simulink model "lqr_hovering"  (R2017a)
settings: Solver=ode5  StartTime=0.0  StopTime=50  FixedStep=Ts  RelTol=1e-3  EnableMultiTasking=on
undefined symbols (not defined in the file or in its folder): B_ENU_inv, gra, Ki_lqr, KT, Kx_lqr, mass
settings Model: Creator=dtnguyen  LastModifiedBy=ducnguyen
settings DataIOCC: LimitDataPoints=on  SaveFormat=Array
settings OptimizationCC: DefaultParameterBehavior=Inlined  UseFloatMulNetSlope=on  InlineInvariantSignals=on  PassReuseOutputArgsThreshold=0  EfficientFloat2IntCast=on
settings DebuggingCC: ParameterTunabilityLossMsg=error  SFUnexpectedBacktrackingDiag=warning  SFNoUnconditionalDefaultTransitionDiag=warning  SFExecutionAtInitializationDiag=none
settings HardwareCC: ProdBitPerPointer=32  ProdBitPerSizeT=32  ProdBitPerPtrDiffT=32  ProdLargestAtomicFloat=None  ProdIntDivRoundTo=Undefined  ProdEndianess=Unspecified  ProdWordSize=32  ProdHWDeviceType=32-bit Generic
settings ModelReferenceCC: PropagateSignalLabelsOutOfModel=off
settings RTWCC: PackageGeneratedCodeAndArtifacts=on  PackageName=myCodeExport  GenerateReport=on  Toolchain=Catkin  BuildConfiguration=Faster Runs  LaunchReport=on  TargetLang=C++  CheckMdlBeforeBuild=Warning
settings CodeAppCC: ForceParamTrailComments=on  OperatorAnnotations=on  MATLABSourceComments=on
settings GRTTargetCC: TargetLangStandard=C++03 (ISO)  MatFileLogging=off  MultiInstanceERTCode=on  CodeInterfacePackaging=C++ class
settings ConfigComp: CovMetricSettings=dw  CovHtmlReporting=on  CovSaveCumulativeToWorkspaceVar=on  CovSaveSingleToWorkspaceVar=on  CovExternalEMLEnable=off

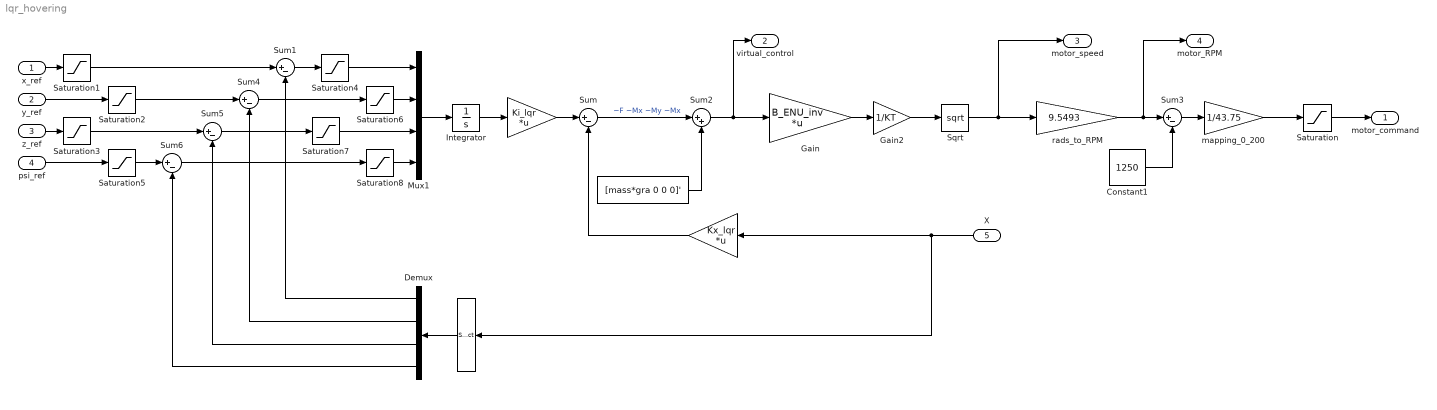
== system lqr_hovering ==
  x_ref : Inport  PortDimensions=1
  y_ref : Inport  Port=2  PortDimensions=1
  z_ref : Inport  Port=3  PortDimensions=1
  psi_ref : Inport  Port=4  PortDimensions=1
  X : Inport  Port=5  PortDimensions=12
  " " : Gain  Gain=Ki_lqr  Multiplication=Matrix(K*u)
  "              " : Constant  Value=[mass*gra 0 0 0]'
  "                   " : Gain  Gain=Kx_lqr  Multiplication=Matrix(K*u)
  "                      " : Selector  InputPortWidth=12  IndexOptions=Index vector (dialog)  Indices=[1 2 3 9]  OutputSizes=1
  Constant1 : Constant  Value=1250  VectorParams1D=off  SampleTime=-1
  Demux : Demux
  Gain : Gain  Gain=B_ENU_inv  Multiplication=Matrix(K*u)
  Gain2 : Gain  Gain=1/KT
  Integrator : Integrator  InitialCondition=[0 0 0 0]'
  Mux1 : Mux
  Saturation : Saturate  UpperLimit=200  LowerLimit=0
  Saturation1 : Saturate  UpperLimit=2  LowerLimit=-2
  Saturation2 : Saturate  UpperLimit=2  LowerLimit=-2
  Saturation3 : Saturate  UpperLimit=1.75  LowerLimit=0
  Saturation4 : Saturate  UpperLimit=1  LowerLimit=-1
  Saturation5 : Saturate  UpperLimit=2*pi  LowerLimit=-2*pi
  Saturation6 : Saturate  UpperLimit=1  LowerLimit=-1
  Saturation7 : Saturate
  Saturation8 : Saturate  UpperLimit=pi/4  LowerLimit=-pi/4
  Sqrt : Sqrt  SaturateOnIntegerOverflow=on
  Sum{,1,3..6} (6 alike) : Sum  Inputs=|+-
  Sum2 : Sum  Inputs=|++
  mapping_0_200 : Gain  Gain=1/43.75
  rads_to_RPM : Gain  Gain=9.5493
  motor_command : Outport  PortDimensions=6
  virtual_control : Outport  Port=2  PortDimensions=4
  motor_speed : Outport  Port=3  PortDimensions=6
  motor_RPM : Outport  Port=4  PortDimensions=6
  wires:
  Gain2/1 -> Sqrt/1
  X/1 -> "                   "/1, "                      "/1
  Mux1/1 -> Integrator/1
  " "/1 -> Sum/1
  Integrator/1 -> " "/1
  "                   "/1 -> Sum/2
  Gain/1 -> Gain2/1
  Sum2/1 -> Gain/1, virtual_control/1
  Sum/1 -> Sum2/1  "~F ~Mx ~My ~Mx"
  "              "/1 -> Sum2/2
  Constant1/1 -> Sum3/2
  rads_to_RPM/1 -> Sum3/1, motor_RPM/1
  Sum3/1 -> mapping_0_200/1
  mapping_0_200/1 -> Saturation/1
  Saturation/1 -> motor_command/1
  z_ref/1 -> Saturation3/1
  x_ref/1 -> Saturation1/1
  y_ref/1 -> Saturation2/1
  Saturation1/1 -> Sum1/1
  Sum1/1 -> Saturation4/1
  Sum4/1 -> Saturation6/1
  Sum5/1 -> Saturation7/1
  Sum6/1 -> Saturation8/1
  "                      "/1 -> Demux/1
  Demux/1 -> Sum1/2
  Demux/2 -> Sum4/2
  Demux/3 -> Sum5/2
  Demux/4 -> Sum6/2
  Saturation2/1 -> Sum4/1
  Saturation3/1 -> Sum5/1
  psi_ref/1 -> Saturation5/1
  Saturation4/1 -> Mux1/1
  Saturation5/1 -> Sum6/1
  Saturation6/1 -> Mux1/2
  Saturation7/1 -> Mux1/3
  Saturation8/1 -> Mux1/4
  Sqrt/1 -> rads_to_RPM/1, motor_speed/1
